simulink model "SP_Robot_Control"  (R2024a)
settings: Solver=VariableStepAuto  StartTime=0.0  StopTime=10.0  RelTol=1e-3
libraries: arduinolib x1, arduinowifilib x1
settings Model: Creator=ammaa  LastModifiedBy=ammaa

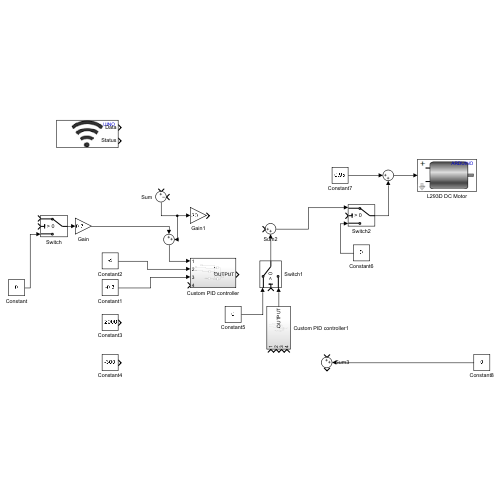
[thumbnail: Simulink's stored preview of the top-level diagram]
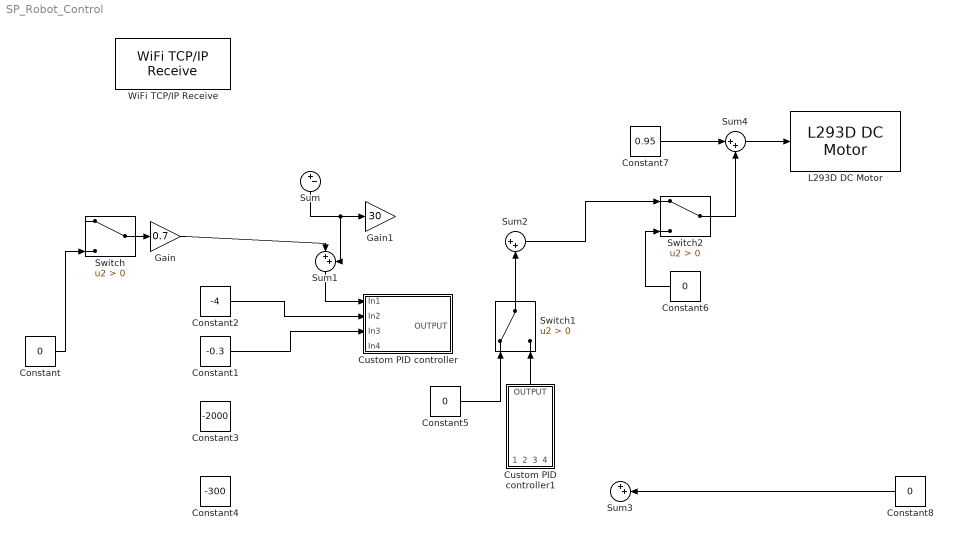
== system SP_Robot_Control ==
  Constant{,5..6,8} (4 alike) : Constant  Value=0
  Constant1 : Constant  Value=-0.3
  Constant2 : Constant  Value=-4
  Constant3 : Constant  Value=-2000
  Constant4 : Constant  Value=-300
  Constant7 : Constant  Value=0.95
  Custom PID controller : Subsystem
  Custom PID controller1 : Subsystem
  Gain : Gain  Gain=0.7
  Gain1 : Gain  Gain=30
  L293D DC Motor : arduinolib/L293D DC Motor  EnablePin=5  InputAPin=8  InputBPin=10
  Sum : Sum  Inputs=|+-
  Sum{1..4} (4 alike) : Sum  Inputs=|++
  Switch : Switch  Criteria=u2 > Threshold  SaturateOnIntegerOverflow=off  InputSameDT=off
  Switch1 : Switch  Criteria=u2 > Threshold  SaturateOnIntegerOverflow=off  InputSameDT=off
  Switch2 : Switch  Criteria=u2 > Threshold  SaturateOnIntegerOverflow=off  InputSameDT=off
  WiFi TCP/IP Receive : arduinowifilib/WiFi TCP//IP Receive  Mode_=Server  serverport=25000  RemoteAddr_=192.168.1.2  RemoteServerPort_=25000  DataType_=uint8  DataSize_=1  SampleTime_=0.1  remoteipoctet1=192  remoteipoctet2=168  remoteipoctet3=1  remoteipoctet4=2  wifiTCPServerIndex=0  wifiTCPClientIndex=0  blockPlatform=ARDUINO  isARMArch=false  BlockingMode_=off  BlockTimeout_=0.1
  wires:
  Switch/1 -> Gain/1
  Constant/1 -> Switch/3
  Sum/1 -> Sum1/2, Gain1/1
  Constant5/1 -> Switch1/1
  Switch1/1 -> Sum2/2
  Sum2/1 -> Switch2/1
  Constant6/1 -> Switch2/3
  Constant8/1 -> Sum3/2
  Gain/1 -> Sum1/1
  Sum1/1 -> Custom PID controller/1(In1)
  Constant2/1 -> Custom PID controller/2(In2)
  Constant1/1 -> Custom PID controller/3(In3)
  Custom PID controller1/1(OUTPUT) -> Switch1/3
  Constant7/1 -> Sum4/1
  Switch2/1 -> Sum4/2
  Sum4/1 -> L293D DC Motor/1

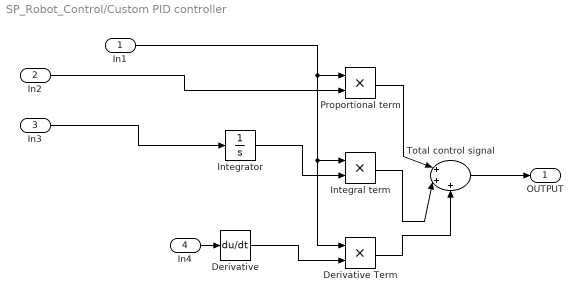
== system SP_Robot_Control/Custom PID controller ==
  In1 : Inport
  In2 : Inport  Port=2
  In3 : Inport  Port=3
  In4 : Inport  Port=4
  Derivative : Derivative
  Derivative Term : Product
  Integral term : Product
  Integrator : Integrator
  Proportional term : Product
  Total control signal : Sum  Inputs=|+++
  OUTPUT : Outport
  wires:
  Total control signal/1 -> OUTPUT/1
  Proportional term/1 -> Total control signal/1
  Integrator/1 -> Integral term/2
  In1/1 -> Derivative Term/1, Integral term/1, Proportional term/1
  Derivative/1 -> Derivative Term/2
  Derivative Term/1 -> Total control signal/3
  Integral term/1 -> Total control signal/2
  In2/1 -> Proportional term/2
  In3/1 -> Integrator/1
  In4/1 -> Derivative/1

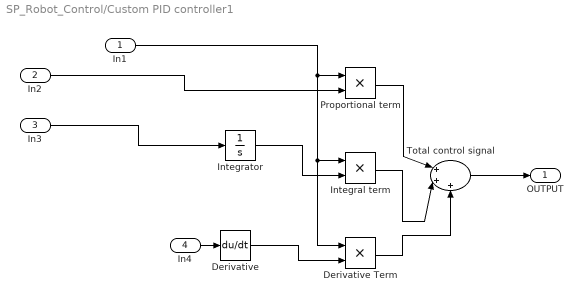
== system SP_Robot_Control/Custom PID controller1 ==
  In1 : Inport
  In2 : Inport  Port=2
  In3 : Inport  Port=3
  In4 : Inport  Port=4
  Derivative : Derivative
  Derivative Term : Product
  Integral term : Product
  Integrator : Integrator
  Proportional term : Product
  Total control signal : Sum  Inputs=|+++
  OUTPUT : Outport
  wires:
  In4/1 -> Derivative/1
  In3/1 -> Integrator/1
  In2/1 -> Proportional term/2
  Integral term/1 -> Total control signal/2
  Derivative Term/1 -> Total control signal/3
  Derivative/1 -> Derivative Term/2
  In1/1 -> Proportional term/1, Integral term/1, Derivative Term/1
  Integrator/1 -> Integral term/2
  Proportional term/1 -> Total control signal/1
  Total control signal/1 -> OUTPUT/1
